simulink model "EX21spectral"  (R2013a)
settings: Solver=ode3  StartTime=0.0  StopTime=2  FixedStep=1.25e-6  RelTol=1e-3
libraries: dsparch4 x1
settings Model: Creator=Dennis Silage  LastModifiedBy=Silage
settings DataIOCC: SignalLoggingSaveFormat=ModelDataLogs
settings OptimizationCC: ExpressionDepthLimit=2147483647  InitFltsAndDblsToZero=on
settings DebuggingCC: FcnCallInpInsideContextMsg=UseLocalSettings  StrictBusMsg=Warning
settings GRTTargetCC: CombineOutputUpdateFcns=off  GRTInterface=on

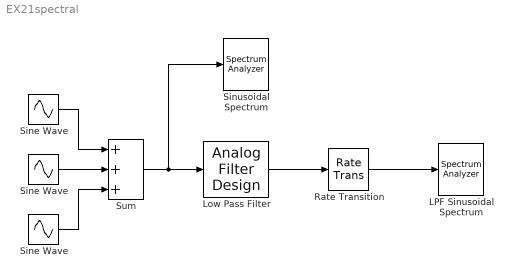
== system EX21spectral ==
  " Sine Wave " : Sin  Amplitude=0.2  Frequency=5000*pi  SampleTime=1.25e-6
  LPF Sinusoidal Spectrum : SpectrumAnalyzer
      settings: CopyFcn=scopeextensions.ScopeBlock.callback(gcbh, 'onBlockCopy', gcbh);  DeleteFcn=scopeextensions.ScopeBlock.callback(gcbh, 'onBlockDelete');  PreSaveFcn=scopeextensions.ScopeBlock.callback(gcbh, 'onModelSave');  NameChangeFcn=scopeextensions.ScopeBlock.callback(gcbh, 'onBlockRename');  CloseFcn=scopeextensions.ScopeBlock.callback(gcbh, 'onBlockClose');  PreDeleteFcn=scopeextensions.ScopeBlock.callback(gcbh, 'onBlockPreDelete');
  Low Pass Filter : dsparch4/Analog Filter Design  method=Butterworth  filttype=Lowpass  N=3  Wlo=pi*2500  Whi=80  Rp=2  Rs=40
  Rate Transition : RateTransition  OutPortSampleTime=1.25e-6
  Sine Wave : Sin  Frequency=1000*pi  SampleTime=1.25e-6
  "Sine Wave " : Sin  Amplitude=0.5  Frequency=3000*pi  SampleTime=1.25e-6
  Sinusoidal Spectrum : SpectrumAnalyzer
      settings: CopyFcn=scopeextensions.ScopeBlock.callback(gcbh, 'onBlockCopy', gcbh);  DeleteFcn=scopeextensions.ScopeBlock.callback(gcbh, 'onBlockDelete');  PreSaveFcn=scopeextensions.ScopeBlock.callback(gcbh, 'onModelSave');  NameChangeFcn=scopeextensions.ScopeBlock.callback(gcbh, 'onBlockRename');  CloseFcn=scopeextensions.ScopeBlock.callback(gcbh, 'onBlockClose');  PreDeleteFcn=scopeextensions.ScopeBlock.callback(gcbh, 'onBlockPreDelete');
  Sum : Sum  Inputs=+++
  wires:
  "Sine Wave "/1 -> Sum/2
  " Sine Wave "/1 -> Sum/3
  Sine Wave/1 -> Sum/1
  Sum/1 -> Sinusoidal Spectrum/1, Low Pass Filter/1
  Low Pass Filter/1 -> Rate Transition/1
  Rate Transition/1 -> LPF Sinusoidal Spectrum/1
